simulink model "arducopter"  (R2021a)
settings: Solver=FixedStepAuto  StartTime=0.0  StopTime=sim.param.timeEnd  FixedStep=sim.param.dt  RelTol=1e-3
undefined symbols (not defined in the file or in its folder): DiscIntNeverNeededParam, sim
libraries: simulink x34, slident x4, vrlib x1
(part 6 of 8)

== system arducopter/Position Controller/set_pos_target_z_from_climb_rate()/input_vel_accel_z/calc accMin ==
  accMax : Inport
  Constant : Constant  Value=750  OutDataTypeStr=single
  Constant1 : Constant  Value=0  OutDataTypeStr=single
  Gain : Gain  Gain=-1
  Saturation Dynamic : simulink/Discontinuities/Saturation Dynamic  OutMin=[]  OutMax=[]  OutDataTypeStr=Inherit: Same as second input  OutDataType=fixdt(1, 16)  OutScaling=2^-10  DoSatur=off
  accMin : Outport
  wires:
  accMax/1 -> Saturation Dynamic/2
  Saturation Dynamic/1 -> Gain/1
  Gain/1 -> accMin/1
  Constant/1 -> Saturation Dynamic/1
  Constant1/1 -> Saturation Dynamic/3

== system arducopter/Position Controller/set_pos_target_z_from_climb_rate()/input_vel_accel_z/shape_vel_accel ==
  note: 1)
  note: shape_vel_accel()
      | Calculates the desired acceleration as a path from the current position, velocity and acceleration to an input velocity, considering the max velocity, acceleration and jerk.
      | Calculate KPa as time constant that defines the error decay in the kinematic path as the system approaches constant acceleration
      | Calculate the preliminary desired acceleration with the square root controller
      | Limit desired acceleration based on max. acceleration and jerk
  note: 3)
  note: 2)
  vel : Inport
  acc : Inport  Port=2
  velDes : Inport  Port=3
  accDes : Inport  Port=4
  accMin : Inport  Port=5
  accMax : Inport  Port=6
  jerkMax : Inport  Port=7
  dt : Inport  Port=8
  limitTotalAccel : Inport  Port=9
  MATLAB Function : MATLAB Function  TreatAsAtomicUnit=on
  Square Root Controller : MATLAB Function  TreatAsAtomicUnit=on
  calc_KPa : MATLAB Function  TreatAsAtomicUnit=on
  accDesShaped : Outport
  wires:
  vel/1 -> calc_KPa/1(velIn)
  acc/1 -> MATLAB Function/4(accIn)
  velDes/1 -> calc_KPa/2(vel)
  accMin/1 -> [accMin]
  accMax/1 -> [accMax]
  jerkMax/1 -> [jerkMax]
  dt/1 -> [dt]
  limitTotalAccel/1 -> MATLAB Function/8(limitTotalAccel)
  calc_KPa/2(KPa) -> Square Root Controller/2(p)
  Square Root Controller/1(correction_rate) -> MATLAB Function/1(accTar)
  MATLAB Function/1(accShaped) -> accDesShaped/1
  accDes/1 -> MATLAB Function/5(acc)
  calc_KPa/1(velErr) -> Square Root Controller/1(err)
  [dt] -> Square Root Controller/4(dt)
  [jerkMax] -> Square Root Controller/3(second_ord_lim)
  [jerkMax] -> calc_KPa/5(jerkMax)
  [dt] -> MATLAB Function/7(dt)
  [jerkMax] -> MATLAB Function/6(jerkMax)
  [accMin] -> calc_KPa/3(accMin)
  [accMax] -> calc_KPa/4(accMax)
  [accMin] -> MATLAB Function/2(accMin)
  [accMax] -> MATLAB Function/3(accMax)

== system arducopter/Position Controller/set_pos_target_z_from_climb_rate()/input_vel_accel_z/update_pos_vel_accel ==
  note: update_pos_vel_accel()
      | Single axis projection of position and velocity forwards in time based on
      | a time step of dt and acceleration off acc.
  posTarIn : Inport
  velDesIn : Inport  Port=2
  accDesIn : Inport  Port=3
  limitVectorZ : Inport  Port=4
  posErr : Inport  Port=5
  velErr : Inport  Port=6
  Constant : Constant  Value=sim.param.dt
  MATLAB Function : MATLAB Function  TreatAsAtomicUnit=on
  posTar : Outport
  velDes : Outport  Port=2
  wires:
  posTarIn/1 -> MATLAB Function/1(posIn)
  velDesIn/1 -> MATLAB Function/2(velIn)
  accDesIn/1 -> MATLAB Function/3(accIn)
  Constant/1 -> MATLAB Function/4(dt)
  MATLAB Function/1(pos) -> posTar/1
  limitVectorZ/1 -> MATLAB Function/5(limit)
  MATLAB Function/2(vel) -> velDes/1
  posErr/1 -> MATLAB Function/6(posErr)
  velErr/1 -> MATLAB Function/7(velErr)

== system arducopter/Rate Controller/PID Pitch Rate/Slew Limiter/Subsystem ==
  p_out : Inport
  d_out : Inport  Port=2
  ATC sample time : Constant  Value=sim.param.dt
  Add : Sum
  Divide : Product  Inputs=*/  OutDataTypeStr=single
  Subtract : Sum  Inputs=+-
  Unit Delay : UnitDelay  InitialCondition=sim.init.PIDP.P+sim.init.PIDP.D  SampleTime=-1  HasFrameUpgradeWarning=on
  sr_raw : Outport
  wires:
  ATC sample time/1 -> Divide/2
  Add/1 -> Unit Delay/1, Subtract/1
  Divide/1 -> sr_raw/1
  p_out/1 -> Add/1
  Unit Delay/1 -> Subtract/2
  Subtract/1 -> Divide/1
  d_out/1 -> Add/2

== system arducopter/Rate Controller/PID Roll Rate/Slew Limiter/Subsystem ==
  p_out : Inport
  d_out : Inport  Port=2
  ATC sample time : Constant  Value=sim.param.dt
  Add : Sum
  Divide : Product  Inputs=*/  OutDataTypeStr=single
  Subtract : Sum  Inputs=+-
  Unit Delay : UnitDelay  InitialCondition=sim.init.PIDR.P + sim.init.PIDR.D  SampleTime=-1  HasFrameUpgradeWarning=on
  sr_raw : Outport
  wires:
  ATC sample time/1 -> Divide/2
  Add/1 -> Unit Delay/1, Subtract/1
  Divide/1 -> sr_raw/1
  p_out/1 -> Add/1
  Unit Delay/1 -> Subtract/2
  Subtract/1 -> Divide/1
  d_out/1 -> Add/2

== system arducopter/Rate Controller/PID Yaw Rate/Slew Limiter/Subsystem ==
  p_out : Inport
  d_out : Inport  Port=2
  ATC sample time : Constant  Value=sim.param.dt
  Add : Sum
  Divide : Product  Inputs=*/  OutDataTypeStr=single
  Subtract : Sum  Inputs=+-
  Unit Delay : UnitDelay  InitialCondition=sim.init.PIDY.P+sim.init.PIDY.D  SampleTime=-1  HasFrameUpgradeWarning=on
  sr_raw : Outport
  wires:
  ATC sample time/1 -> Divide/2
  Add/1 -> Unit Delay/1, Subtract/1
  Divide/1 -> sr_raw/1
  p_out/1 -> Add/1
  Unit Delay/1 -> Subtract/2
  Subtract/1 -> Divide/1
  d_out/1 -> Add/2

== system arducopter/Attitude Controller/input_euler_angle_roll_pitch_euler_rate_yaw()/Feedforward enabled/input shaping/input shaping pitch angle ==
  note: AC_AttitudeControl::input_shaping_angle(float error_angle, float input_tc, float accel_max, float target_ang_vel, float desired_ang_vel, float max_ang_vel, float dt)
      | Calculation of velocity correction from an angle error. The angular velocity has acceleration and deceleration limits including basic jerk limiting using _input_tc.
      |
      | Function is called from input_shaping_angle(float error_angle, float smoothing_gain, float accel_max, float target_ang_vel, float dt) as input_shaping_angle(error_angle, smoothing_gain, accel_max, target_ang_vel, 0.0f, 0.0f, dt), so desired_ang_vel = 0 and max_ang_vel = 0
  pitchAngleErr : Inport
  pitchRateTarIn : Inport  Port=2
  pitchAccelMax : Inport  Port=3
  Constant : Constant  Value=sim.param.dt  VectorParams1D=off
  Constant1 : Constant  Value=sim.param.ATC.INPUT_TC  VectorParams1D=off
  Constant2 : Constant  Value=sim.param.dt  VectorParams1D=off
  Data Type Conversion : DataTypeConversion  OutDataTypeStr=single
  Data Type Conversion1 : DataTypeConversion  OutDataTypeStr=single
  MATLAB Function : MATLAB Function  TreatAsAtomicUnit=on
  MATLAB Function1 : MATLAB Function  TreatAsAtomicUnit=on
  Square Root Controller : MATLAB Function  TreatAsAtomicUnit=on
  calc p from input_tc : Subsystem
  eulerPitchRateTar : Outport
  wires:
  MATLAB Function1/1(eulerRateTar) -> eulerPitchRateTar/1
  [accelMax] -> MATLAB Function1/3(accelMax)
  [accelMax] -> Square Root Controller/3(second_ord_lim)
  Constant2/1 -> Data Type Conversion1/1
  Square Root Controller/1(correction_rate) -> MATLAB Function1/1(desiredAngVel)
  calc p from input_tc/1(p) -> Square Root Controller/2(p)
  Constant1/1 -> calc p from input_tc/1(input_tc)
  Constant/1 -> Data Type Conversion/1
  pitchAccelMax/1 -> [accelMax]
  MATLAB Function/1(radLim) -> Square Root Controller/1(err)
  pitchAngleErr/1 -> MATLAB Function/1(radIn)
  pitchRateTarIn/1 -> MATLAB Function1/2(targetAngVel)
  Data Type Conversion/1 -> Square Root Controller/4(dt)
  Data Type Conversion1/1 -> MATLAB Function1/4(dt)

== system arducopter/Attitude Controller/input_euler_angle_roll_pitch_euler_rate_yaw()/Feedforward enabled/input shaping/input shaping roll angle ==
  note: AC_AttitudeControl::input_shaping_angle(float error_angle, float input_tc, float accel_max, float target_ang_vel, float desired_ang_vel, float max_ang_vel, float dt)
      | Calculation of velocity correction from an angle error. The angular velocity has acceleration and deceleration limits including basic jerk limiting using _input_tc.
      |
      | Function is called from input_shaping_angle(float error_angle, float smoothing_gain, float accel_max, float target_ang_vel, float dt) as input_shaping_angle(error_angle, smoothing_gain, accel_max, target_ang_vel, 0.0f, 0.0f, dt), so desired_ang_vel = 0 and max_ang_vel = 0
  rollAngleErr : Inport
  rollRateTarIn : Inport  Port=2
  rollAccelMax : Inport  Port=3
  Constant : Constant  Value=sim.param.dt  VectorParams1D=off
  Constant1 : Constant  Value=sim.param.ATC.INPUT_TC  VectorParams1D=off
  Constant2 : Constant  Value=sim.param.dt  VectorParams1D=off
  Data Type Conversion : DataTypeConversion  OutDataTypeStr=single
  Data Type Conversion1 : DataTypeConversion  OutDataTypeStr=single
  MATLAB Function : MATLAB Function  TreatAsAtomicUnit=on
  MATLAB Function1 : MATLAB Function  TreatAsAtomicUnit=on
  Square Root Controller : MATLAB Function  TreatAsAtomicUnit=on
  calc p from input_tc : Subsystem
  eulerRollRateTar : Outport
  wires:
  rollAngleErr/1 -> MATLAB Function/1(radIn)
  MATLAB Function/1(radLim) -> Square Root Controller/1(err)
  rollAccelMax/1 -> [accelMax]
  Constant/1 -> Data Type Conversion/1
  Constant1/1 -> calc p from input_tc/1(input_tc)
  calc p from input_tc/1(p) -> Square Root Controller/2(p)
  Square Root Controller/1(correction_rate) -> MATLAB Function1/1(desiredAngVel)
  Constant2/1 -> Data Type Conversion1/1
  [accelMax] -> Square Root Controller/3(second_ord_lim)
  [accelMax] -> MATLAB Function1/3(accelMax)
  MATLAB Function1/1(eulerRateTar) -> eulerRollRateTar/1
  rollRateTarIn/1 -> MATLAB Function1/2(targetAngVel)
  Data Type Conversion/1 -> Square Root Controller/4(dt)
  Data Type Conversion1/1 -> MATLAB Function1/4(dt)

== system arducopter/Attitude Controller/input_euler_angle_roll_pitch_euler_rate_yaw()/Feedforward enabled/input shaping/input shaping yaw rate ==
  note: AC_AttitudeControl::input_shaping_ang_vel()
      | Limits the maximum acceleration resulting from the target yaw rate, so that the target yaw rate is slewed towards the input rate
  yawRateDes : Inport
  yawRateTar : Inport  Port=2
  eulerAccelMax : Inport  Port=3
  Constant2 : Constant  Value=sim.param.dt  VectorParams1D=off
  Data Type Conversion : DataTypeConversion  OutDataTypeStr=single
  MATLAB Function1 : MATLAB Function  TreatAsAtomicUnit=on
  eulerYawRateTar : Outport
  wires:
  yawRateDes/1 -> MATLAB Function1/1(desiredAngVel)
  Constant2/1 -> Data Type Conversion/1
  eulerAccelMax/1 -> MATLAB Function1/3(accelMax)
  MATLAB Function1/1(eulerRateTar) -> eulerYawRateTar/1
  yawRateTar/1 -> MATLAB Function1/2(targetAngVel)
  Data Type Conversion/1 -> MATLAB Function1/4(dt)

== system arducopter/Attitude Controller/input_euler_angle_roll_pitch_euler_rate_yaw()/thrust_heading_rotation_angles()/Yaw error limitation/Yaw limiting and recalculation of attitudeTarget ==
  note: Limit yaw error and calculate new attitudeTarget and attitudeError
  note: Create new attitudeError with limited yaw error
  note: Calculate new attitudeTarget with limited yawVecCorrection
  note: Limit yaw error based on maximum acceleration
  attitudeErrorIn : Inport
  thrustVecCorrection : Inport  Port=2
  attitudeBody : Inport  Port=3
  Enable : EnablePort
  Constant : Constant  Value=sim.param.ATC.ACCEL_Y_CONTROLLER_MAX_RADSS
  Constant1 : Constant  Value=sim.param.ATC.ANG_YAW_P
  Constant2 : Constant  Value=0  OutDataTypeStr=single
  Demux : Demux  Outputs=2
  Divide : Product  Inputs=*/
  Gain : Gain  Gain=-1
  MATLAB Function : MATLAB Function  TreatAsAtomicUnit=on
  MATLAB Function1 : MATLAB Function  TreatAsAtomicUnit=on
  MATLAB Function5 : MATLAB Function  TreatAsAtomicUnit=on
  MATLAB Function9 : MATLAB Function  TreatAsAtomicUnit=on
  MinMax : MinMax  Inputs=2
  MinMax1 : MinMax  Function=max  Inputs=2
  Mux : Mux  Inputs=3
  Mux1 : Mux  Inputs=3
  Selector : Selector  InputPortWidth=3  IndexOptions=Index vector (dialog)  Indices=[3]  OutputSizes=1
  Selector1 : Selector  InputPortWidth=3  IndexOptions=Index vector (dialog)  Indices=[1 2]  OutputSizes=1
  attitudeTarget : Outport
  attitudeError : Outport  Port=2
  wires:
  Constant/1 -> Divide/1
  Constant1/1 -> Divide/2
  [attitudeError] -> Selector/1
  Selector/1 -> MinMax/1
  Divide/1 -> MinMax/2, Gain/1
  MinMax/1 -> MinMax1/1
  Gain/1 -> MinMax1/2
  MinMax1/1 -> MATLAB Function/1(radIn)
  MATLAB Function/1(radLim) -> Mux1/3, Mux/3
  Constant2/1 -> Mux/2, Mux/1
  Mux/1 -> MATLAB Function5/1(vec)
  MATLAB Function5/1(q) -> MATLAB Function9/2(q2)  "yawVecCorrection"
  MATLAB Function9/1(qRes) -> MATLAB Function1/2(q2)
  thrustVecCorrection/1 -> MATLAB Function9/1(q1)
  attitudeBody/1 -> MATLAB Function1/1(q1)
  MATLAB Function1/1(qRes) -> attitudeTarget/1
  Mux1/1 -> attitudeError/1
  attitudeErrorIn/1 -> [attitudeError]
  [attitudeError] -> Selector1/1
  Selector1/1 -> Demux/1
  Demux/1 -> Mux1/1
  Demux/2 -> Mux1/2

== system arducopter/Attitude Controller/input_euler_angle_roll_pitch_euler_rate_yaw()/Feedforward enabled/input shaping/input shaping pitch angle/calc p from input_tc ==
  note: Calculation of proportional factor of square root controller.
      | Based on function argument of sqrt_controller() in AC_AttitudeControl::input_shaping_angle()
  input_tc : Inport
  Constant2 : Constant  Value=0.01  OutDataTypeStr=single
  Constant3 : Constant  OutDataTypeStr=single
  Divide : Product  Inputs=*/
  Max : MinMax  Function=max  Inputs=2
  p : Outport
  wires:
  Constant2/1 -> Max/2
  Max/1 -> Divide/2
  Constant3/1 -> Divide/1
  input_tc/1 -> Max/1
  Divide/1 -> p/1

== system arducopter/Attitude Controller/input_euler_angle_roll_pitch_euler_rate_yaw()/Feedforward enabled/input shaping/input shaping roll angle/calc p from input_tc ==
  note: Calculation of proportional factor of square root controller.
      | Based on function argument of sqrt_controller() in AC_AttitudeControl::input_shaping_angle()
  input_tc : Inport
  Constant2 : Constant  Value=0.01  OutDataTypeStr=single
  Constant3 : Constant  OutDataTypeStr=single
  Divide : Product  Inputs=*/
  Max : MinMax  Function=max  Inputs=2
  p : Outport
  wires:
  Constant2/1 -> Max/2
  Max/1 -> Divide/2
  Constant3/1 -> Divide/1
  input_tc/1 -> Max/1
  Divide/1 -> p/1

== matlab function arducopter/Position Controller/set z component of limit vec/MATLAB Function ==
function limVecZ = fcn(limLower, limUpper)
% Based on AC_PosControl::update_z_controller()

if limUpper
    limVecZ = single(1);
elseif limLower
    limVecZ = single(-1);
else
    limVecZ = single(0);
end

== matlab function arducopter/Throttle/Throttle Calculations/Throttle Hover/Throttle Hover Calculation ==
function thrHover = updateThrHov(dt, thrAct, zVelDes, zVelAct, thstHoverMax, thstHoverMin, thstHoverTC, thstHoverDefault, hoverLearn, thrMan)
%% Code is based on Copter::update_throttle_hover() in Attitude.cpp

global thrHoverAct;

% Use default throttle hover when throttle is set to manual
if (thrMan)
    thrHoverAct = thstHoverDefault;
end
if zVelDes > 0
    thrHoverAct = thstHoverDefault;
end

% Calc average throttle if we are in level hpver
if (thrAct > 0  && abs(zVelAct) < 60)
    %% Code is based on AP_MotorsMulticopter::update_throttle_hover(dt) in AP_MotorsMulticopter.cpp
    % Update throttle hover in dependency of the current output throttle
    if ( (hoverLearn ~= 0))
        thrHoverAct = thrHoverAct + (dt / (dt + thstHoverTC) ) * (thrAct - thrHoverAct);

        % Limit throttle hover to specified limits
        thrHoverAct = max( min( thrHoverAct, thstHoverMax), thstHoverMin);
    else % Set hover to default value if learning is disabled (AP_MotorsMulticopter.cpp)
        thrHoverAct = thstHoverDefault;
    end
end

thrHover = thrHoverAct;

== matlab function arducopter/Position Controller/set_pos_target_z_from_climb_rate()/input_vel_accel_z/shape_vel_accel/calc_KPa ==
function [velErr, KPa] = calcKPa(velIn, vel, accMin, accMax, jerkMax)
% First part of shape_vel_accel() in control.cpp
% Calculates correction gain KPa for the square root controller based on
% the jerk and acceleration limits.

% Velocity error to be corrected
velErr = velIn - vel;

% Calculate time constants and limits to ensure stable operation.
% The direction of acceleration limit is the same as the velocity error.
% This is because the velocity error is negative when slowing down while
% closing a positive position error.
if velErr > 0
    KPa = jerkMax / accMax;
else
    KPa = jerkMax / (-accMin);
end

== matlab function arducopter/Position Controller/set_pos_target_z_from_climb_rate()/input_vel_accel_z/shape_vel_accel/Square Root Controller ==
function correction_rate = sqrt_controller(err, p, second_ord_lim, dt)
% The square root controller
% Code is taken from sqrt_controller(...) in AC_PosControl.cpp.

if (second_ord_lim < 0 || second_ord_lim == 0)
   correction_rate = err * p;
elseif (p == 0)
    % P term is zero, but second order limit is positive
    if (err > 0)
        correction_rate = sqrt(single(2.0) * second_ord_lim * err);
    elseif (err < 0)
        correction_rate = sqrt(single(2.0) * second_ord_lim * -err);
    else
        correction_rate = single(0.0);
    end
else
    % P term and second order limit are positive, hence have been defined
    linear_dist = second_ord_lim / (p * p);
    % Check if error exceeds linear range of controller gain
    if (err > linear_dist)
        correction_rate = sqrt(single(2.0) * second_ord_lim * ( err - (linear_dist / single(2.0)) ));
    elseif (err < -linear_dist)
        correction_rate = -sqrt(single(2.0) * second_ord_lim * ( -err - (linear_dist / single(2.0)) ));
    else
        % Return linearly amplified correction if error is in linear range
        correction_rate = err * p;
    end
end

% Prevent oscillations by over-shooting the error correction in the last
% time step
if (dt ~= 0)
    correction_rate = max( min(correction_rate, abs(err) / dt), -abs(err) / dt);
end

== matlab function arducopter/Position Controller/set_pos_target_z_from_climb_rate()/input_vel_accel_z/shape_vel_accel/MATLAB Function ==
function accShaped = shapeAccelDes(accTar, accMin, accMax, accIn, acc, jerkMax, dt, limitTotalAccel)
% Second part of shape_vel_accel() in control.cpp
% Constrains desired acceleration based on acceleration limits and shapes
% kinematic path according to max jerk

%% 1) Limit desired acceleration based on acceleration limits
% Constrain correction acceleration from accMin to accMax
accTar = max(min(accTar, accMax), accMin);

% Velocity correction with input velocity
accTar = accTar + accIn;

% Constrain total acceleration from accMin to accMax
if limitTotalAccel
    accTar = max(min(accTar, accMax), accMin);
end

%% 2) Calculate required jerk limited adjustment to the current acceleration
% for the next time dt. Based on shape_accel()
accDelta = accTar - acc;
if jerkMax > 0
    accDelta = max(min(accDelta, jerkMax*dt), -jerkMax*dt);
end
accShaped = acc + accDelta;

== matlab function arducopter/Position Controller/get_pilot_speed_dn()/MATLAB Function ==
function dnMax = getPilotSpeedDown(dnMaxIn, upMax)
% Get maximum vertical descending velocity. Called in ModeAltHold::init()
% in the function call for AC_PosControl::set_max_speed_accel_z()
if dnMaxIn == 0
    dnMax = abs(upMax);
else
    dnMax = abs(dnMaxIn);
end

== matlab function arducopter/Throttle/Throttle Calculations/Throttle Limiting based on battery state/Update Lift Max from Battery Voltage ==
function [battVoltFilt, liftMax, battVoltMinAct, battVoltRestEstAct] = fcn(battVoltFiltLast, battVoltRestEst, battVoltMax, battVoltMin, thstCurveExpo, loop_rate)
% Code taken from AP_MotorsMulticopter::update_lift_max_from_batt_voltage()
% in AP_MotorsMulticopter.cpp

% Check if batt_volt_min is too small
if (battVoltMax <= 0 || (battVoltMin >= battVoltMax) ...
        || battVoltRestEst < 0.25 * battVoltMin)
    battVoltFilt = single(1.0);
    liftMax = single(1.0);
    battVoltMinAct = battVoltMin;
    battVoltRestEstAct = battVoltRestEst;
    return;
end

% Set lower battery voltage limit for thrust scaling to a new value
battVoltMinAct = max(battVoltMin, battVoltMax * 0.6);

% Constrain resting voltage estimate (resting voltage is actual voltage
% with sag removed based on current draw and resistance)
battVoltRestEstAct = max( min(battVoltRestEst, battVoltMax), battVoltMin);

%% Filter battery voltage at 0.5 Hz. 
% Cutoff Frequency defined in AP_MotorsMulticopter.h
cutoff_freq = single(0.5);
% Calculate time constant and alpha value
T = 1 / (2 * pi * cutoff_freq);
dt = 1 / loop_rate;
alpha = dt / (dt + T);
alpha = max( min( alpha, 1.0), 0.0);

% Filter input is batt_volt_rest_est / batt_volt_comp_max
in = battVoltRestEstAct / battVoltMax;

% Output calculation
battVoltFilt = battVoltFiltLast + (in - battVoltFiltLast) * alpha;

%% Calculate lift_max
thstCurveExpo = max( min(thstCurveExpo, 1), -1);
liftMax = battVoltFilt * (1 - thstCurveExpo) + thstCurveExpo * battVoltFilt * battVoltFilt;

== matlab function arducopter/Throttle/Throttle Calculations/Throttle Limiting based on battery state/Get current throttle limit ==
function [thrThstMax, thrLimit] = getCurrentLimitMaxThrottle(batVoltMin, batCurrMax, batCurrT, loop_rate, batCurr, batRes, batVolt, thrHover, thrLimitLast)
% Code is based on AP_MotorsMulticopter::get_current_limit_max_throttle()
% in AP_MotorsMulticopter.cpp. 
% Returns a throttle limit based on the maximum battery current as a number
% from 0~1 in the range throttle_min to throttle_max.

% Return maximum if current limiting is disabled
if(batCurrMax <= 0) 
    thrLimit = single(1.0);
    thrThstMax = single(1.0);
    return;
end
% Return maximum if battery resistance is not measured
if(batRes == 0)
    thrLimit = single(1.0);
    thrThstMax = single(1.0);
    return;
end

%% Calculate throttle limit
% The throttle limit represents the maximum throttle potential that is left
% based on the actual current compared to the maximum battery current.

% Maximum current to prevent voltage sag below batt_voltage_min
% Since the actual battery current level is used as the minimum for the limit,
% the actual current can still be used to maintain the current throttle. 
batt_curr_max_new = min(batCurrMax, batCurr + (batVolt - batVoltMin) / batRes);
% Calcualte current artion
batt_curr_ratio = batCurr / batt_curr_max_new;
% Calculate time step
dt = 1 / loop_rate;
% Calculate throttle limit as the additional throttle on top of throttle
% hover
thrLimit = thrLimitLast + (dt / (dt + batCurrT)) * (1.0 - batt_curr_ratio);
% Throttle limit drops to 20% between hover an full throttle
thrLimit = max( min( thrLimit, 1.0), 0.2);

% Calculate maximum throttle as sum of hover throttle and the possible
% additional throttle based on the maximum current.
thrThstMax = thrHover + ((1.0 - thrHover) * thrLimit);

== matlab function arducopter/Rate Controller/PID Yaw Rate/I/Integrator ==
function integrator_out = fcn(error, integrator, limit_flg, ki, i_max, dt)
% Code is based on AC_PID::update_i() in AC_PID.cpp.

% Check plausibility of input parameters
if (ki ~= 0 && dt > 0)
    % Only allow integration if limit is not set or the absolute sum of the
    % integrator would be reduced.
    if (~limit_flg || (integrator > 0 && error < 0) || (integrator < 0 && error > 0))
        integrator_out = integrator + error * ki * dt;
        integrator_out = max( min(integrator_out, i_max), -i_max);
    else % Otherwise, keep old integrator value
        integrator_out = integrator;
    end
else % Reset integrator if input parameters are not plausible
    integrator_out = single(0.0);
end

== matlab function arducopter/Rate Controller/PID Roll Rate/I/Integrator ==
function integrator_out = fcn(error, integrator, limit_flg, ki, i_max, dt)
% Code is based on AC_PID::update_i() in AC_PID.cpp.

% Check plausibility of input parameters
if (ki ~= 0 && dt > 0)
    % Only allow integration if limit is not set or the absolute sum of the
    % integrator would be reduced.
    if (~limit_flg || (integrator > 0 && error < 0) || (integrator < 0 && error > 0))
        integrator_out = integrator + error * ki * dt;
        integrator_out = max( min(integrator_out, i_max), -i_max);
    else % Otherwise, keep old integrator value
        integrator_out = integrator;
    end
else % Reset integrator if input parameters are not plausible
    integrator_out = single(0.0);
end

== matlab function arducopter/Throttle/Throttle Calculations/Get compensation gain ==
function compGain = fcn(liftMax, airDensityRatio)
% Code is based on AP_MotorsMulticopter::get_compensation_gain() in
% AP_MotorsMulticopter.cpp.

% Avoid to divide by zero
if(liftMax <= 0.0)
    compGain = single(1.0);
    return;
end

compGain = 1.0 / liftMax;

% Limit air density ratio
airDensityRatioLim = double(max( min( airDensityRatio, 1.25 ), 0.5));

if (airDensityRatio > 0.3 && airDensityRatio < 1.5)
   compGain = compGain * (1.0 / airDensityRatioLim); 
end

== matlab function arducopter/Rate Controller/PID Roll Rate/Slew Limiter/Calculate Dmod ==
function Dmod   = fcn(slew_rate, sr_max, sr_tau, dt, time)
% Code is based on SlewLimiter::modifier() in SlewLimiter.cpp. 

% Define global variables, so that quanitities do not have to be fed back
% to the function
global pos_event_stored;
global pos_event_idx;
global pos_event_ms;
global max_pos_slew_rate;
global max_pos_slew_event_ms;
global neg_event_stored;
global neg_event_idx;
global neg_event_ms;
global max_neg_slew_rate;
global max_neg_slew_event_ms;
global modifier_slew_rate;
global output_slew_rate;

% Definition of constants as done in SlewLimiter.h
N_EVENTS = uint32(3); % Number of positive and negative consecutive slew rate exceedance events recorded. Set to 3 because of 1-based indexing.
WINDOW_MS = uint32(300); % Time in ms required for half a cycle of the slowest oscillation frequency expected
MODIFIER_GAIN = 1.5; % Ratio of modifier reduction to slew rate exceedance

% Check if slew limiter is activated
if(sr_max <= 0)
   Dmod = single(1.0);
end

now_ms = uint32(time);
decay_alpha = min(dt, sr_tau) / sr_tau;

%% Save exceedance events in event time vector
% Store a series of positive slew rate exceedance events
if (~pos_event_stored && slew_rate > sr_max)
    if (pos_event_idx >= N_EVENTS)
        pos_event_idx(:) = 1;
    end
    pos_event_ms(pos_event_idx) = now_ms;
    pos_event_idx(:) = pos_event_idx + 1;
    pos_event_stored = true;
    neg_event_stored = false;
end

% Store a series of negative slew rate exceedance events
if (~neg_event_stored && slew_rate < -sr_max)
    if (neg_event_idx >= N_EVENTS)
        neg_event_idx(:) = 1;
    end
    neg_event_ms(neg_event_idx) = now_ms;
    neg_event_idx(:) = neg_event_idx + 1;
    pos_event_stored = false;
    neg_event_stored = true;
end

% Find oldest event time
oldest_ms = now_ms;
for i=1:N_EVENTS-1
   if (pos_event_ms(i) < oldest_ms)
       oldest_ms = pos_event_ms(i);
   end
   if (neg_event_ms(i) < oldest_ms)
       oldest_ms = neg_event_ms(i);
   end
end

%% Calculate maximum slew rate
% Save new maximum slew rates, if oldest maximum is exceeded
% OR decay the peak slew rates (pos. and neg.) if they are outside the
% observed time window
if (slew_rate > max_pos_slew_rate)
    max_pos_slew_rate(:) = min(slew_rate, 10 * sr_max);
    max_pos_slew_event_ms = now_ms;
elseif (now_ms - max_pos_slew_event_ms > WINDOW_MS)
    max_pos_slew_rate = max_pos_slew_rate * (1.0 - decay_alpha);
end

if (slew_rate < -max_neg_slew_rate)
    max_neg_slew_rate(:) = min(-slew_rate, 10 * sr_max);
    max_neg_slew_event_ms = now_ms;
elseif (now_ms - max_neg_slew_event_ms > WINDOW_MS)
    max_neg_slew_rate = max_neg_slew_rate * (1.0 - decay_alpha);
end

% Calculate the averaged maximum slew rate
raw_slew_rate = 0.5 * (max_pos_slew_rate + max_neg_slew_rate);

% When the oldest exceedance event falls outside of the window required for
% the number of exceedance events, apply a further reduction to the maximum
% slew rate. This prevents unwanted gain reductions caused by spikes in the
% demanded angular rates due to changed control modes or similar causes.
modifier_input = raw_slew_rate;
if(now_ms - oldest_ms > N_EVENTS * WINDOW_MS) % no incrementation of N_EVENTS because of 1 based indexing
   oldest_time_from_window = single(0.001) * single(now_ms - oldest_ms - N_EVENTS * WINDOW_MS); 
   modifier_input = modifier_input * single(exp(-oldest_time_from_window / sr_tau));
end

%% Calculation of modifier and output slew rate

% Apply filter to slew rate in order to reduce effects of large setpoint
% changes
attack_alpha = min(2.0 * decay_alpha, 1.0);

modifier_slew_rate = modifier_slew_rate + (modifier_input - modifier_slew_rate) * attack_alpha;
modifier_slew_rate = min(modifier_slew_rate, modifier_input);

output_slew_rate = output_slew_rate + (raw_slew_rate - output_slew_rate) * attack_alpha;
output_slew_rate = min(raw_slew_rate, output_slew_rate);

% Calculate modifier. Only has an impact if sr_max is exceeded by averaged
% slew rate.
if(modifier_slew_rate > sr_max)
    Dmod(:) = sr_max / (sr_max + MODIFIER_GAIN * (modifier_slew_rate - sr_max));
else
    Dmod(:) = 1.0;
end

== matlab function arducopter/Rate Controller/PID Roll Rate/Slew Limiter/Lowpass Filter ==
function out  = fcn(in, cutoff_freq, loop_rate, out_last)
% The code is based on the apply(sample, cutoff_freq, dt) function in
% LowPassFilter.cpp
dt = 1 / loop_rate;

% Check if filter is supposed to be filtering
if (cutoff_freq <=0 || dt <= 0)
    out = in;
    return;
end

% Calculate time constant and alpha value
T = 1 / (2 * pi * cutoff_freq);
alpha = dt / (dt + T);
alpha = max( min( alpha, 1.0), 0.0);

% Output calculation
out = out_last + (in - out_last) * alpha;

== matlab function arducopter/Throttle/Throttle Calculations/Air density Calculation/Get equivalent to true airspeed EAS2TAS ==
function eas2tas = fcn(alt, airPress, gndTemp)
% Code is based on AP_Baro::get_EAS2TAS() in AP_Baro.cpp.

% Constants
C_TO_KELVIN = single(273.15); % Conversion offset from celsius to kelvin
ISA_LAPSE_RATE = single(0.0065);
ISA_GAS_CONSTANT = single(287.26);
SSL_AIR_DENSITY = single(1.225);

% Global variables
global EAS2TAS;
global last_alt_EAS2TAS;

% Check if altitude has changed significally
if ((abs(alt - last_alt_EAS2TAS) < 25.0) && EAS2TAS ~= 0)
    % Change too small to require re-calculating
   eas2tas = EAS2TAS;
   return;
end

if (airPress == 0)
   eas2tas = single(1.0);
   return;
end

tempK = single(gndTemp + C_TO_KELVIN - ISA_LAPSE_RATE * alt);
eas2tas_squared = SSL_AIR_DENSITY / (airPress / (ISA_GAS_CONSTANT * tempK));
if (eas2tas_squared <= 0)
    eas2tas = single(1.0);
    return;
end
EAS2TAS = sqrt(eas2tas_squared);
last_alt_EAS2TAS = alt;
eas2tas = EAS2TAS;

== matlab function arducopter/Throttle/Throttle Calculations/Air density Calculation/Get air density ratio ==
function airDensityRatio = fcn(eas2tas)
% Code is based on AP_Baro::get_air_density_ratio() in AP_Baro.cpp.
if (eas2tas > 0.0)
    airDensityRatio = single(1.0 / (eas2tas*eas2tas));
else
    airDensityRatio = single(1.0);
end

== matlab function arducopter/Attitude Controller/input_euler_angle_roll_pitch_euler_rate_yaw()/Feedforward enabled/input shaping/input shaping pitch angle/MATLAB Function1 ==
function eulerRateTar = input_shaping_ang_vel(desiredAngVel, targetAngVel, accelMax, dt)
% Limits acceleration and deceleration of a velocity request
% Code based on AC_AttitudeControl::input_shaping_ang_vel()

% Acceleration is limited directly to smooth the beginning of the curve
if accelMax > 0
    deltaAngVel = accelMax * dt;
    eulerRateTar = min(max(desiredAngVel, targetAngVel - deltaAngVel), targetAngVel + deltaAngVel);
else
    eulerRateTar = desiredAngVel;
end

== matlab function arducopter/Attitude Controller/input_euler_angle_roll_pitch_euler_rate_yaw()/Feedforward enabled/input shaping/input shaping yaw rate/MATLAB Function1 ==
function eulerRateTar = input_shaping_ang_vel(desiredAngVel, targetAngVel, accelMax, dt)
% Limits acceleration and deceleration of a velocity request
% Code based on AC_AttitudeControl::input_shaping_ang_vel()

% Acceleration is limited directly to smooth the beginning of the curve
if accelMax > 0
    deltaAngVel = accelMax * dt;
    eulerRateTar = min(max(desiredAngVel, targetAngVel - deltaAngVel), targetAngVel + deltaAngVel);
else
    eulerRateTar = desiredAngVel;
end

== matlab function arducopter/Rate Controller/PID Yaw Rate/Slew Limiter/Calculate Dmod ==
function Dmod   = fcn(slew_rate, sr_max, sr_tau, dt, time)
% Code is based on SlewLimiter::modifier() in SlewLimiter.cpp. 

% Define global variables, so that quanitities do not have to be fed back
% to the function
global pos_event_stored;
global pos_event_idx;
global pos_event_ms;
global max_pos_slew_rate;
global max_pos_slew_event_ms;
global neg_event_stored;
global neg_event_idx;
global neg_event_ms;
global max_neg_slew_rate;
global max_neg_slew_event_ms;
global modifier_slew_rate;
global output_slew_rate;

% Definition of constants as done in SlewLimiter.h
N_EVENTS = uint32(3); % Number of positive and negative consecutive slew rate exceedance events recorded. Set to 3 because of 1-based indexing.
WINDOW_MS = uint32(300); % Time in ms required for half a cycle of the slowest oscillation frequency expected
MODIFIER_GAIN = 1.5; % Ratio of modifier reduction to slew rate exceedance

% Check if slew limiter is activated
if(sr_max <= 0)
   Dmod = single(1.0);
end

now_ms = uint32(time);
decay_alpha = min(dt, sr_tau) / sr_tau;

%% Save exceedance events in event time vector
% Store a series of positive slew rate exceedance events
if (~pos_event_stored && slew_rate > sr_max)
    if (pos_event_idx >= N_EVENTS)
        pos_event_idx(:) = 1;
    end
    pos_event_ms(pos_event_idx) = now_ms;
    pos_event_idx(:) = pos_event_idx + 1;
    pos_event_stored = true;
    neg_event_stored = false;
end

% Store a series of negative slew rate exceedance events
if (~neg_event_stored && slew_rate < -sr_max)
    if (neg_event_idx >= N_EVENTS)
        neg_event_idx(:) = 1;
    end
    neg_event_ms(neg_event_idx) = now_ms;
    neg_event_idx(:) = neg_event_idx + 1;
    pos_event_stored = false;
    neg_event_stored = true;
end

% Find oldest event time
oldest_ms = now_ms;
for i=1:N_EVENTS-1
   if (pos_event_ms(i) < oldest_ms)
       oldest_ms = pos_event_ms(i);
   end
   if (neg_event_ms(i) < oldest_ms)
       oldest_ms = neg_event_ms(i);
   end
end

%% Calculate maximum slew rate
% Save new maximum slew rates, if oldest maximum is exceeded
% OR decay the peak slew rates (pos. and neg.) if they are outside the
% observed time window
if (slew_rate > max_pos_slew_rate)
    max_pos_slew_rate(:) = min(slew_rate, 10 * sr_max);
    max_pos_slew_event_ms = now_ms;
elseif (now_ms - max_pos_slew_event_ms > WINDOW_MS)
    max_pos_slew_rate = max_pos_slew_rate * (1.0 - decay_alpha);
end

if (slew_rate < -max_neg_slew_rate)
    max_neg_slew_rate(:) = min(-slew_rate, 10 * sr_max);
    max_neg_slew_event_ms = now_ms;
elseif (now_ms - max_neg_slew_event_ms > WINDOW_MS)
    max_neg_slew_rate = max_neg_slew_rate * (1.0 - decay_alpha);
end

% Calculate the averaged maximum slew rate
raw_slew_rate = 0.5 * (max_pos_slew_rate + max_neg_slew_rate);

% When the oldest exceedance event falls outside of the window required for
% the number of exceedance events, apply a further reduction to the maximum
% slew rate. This prevents unwanted gain reductions caused by spikes in the
% demanded angular rates due to changed control modes or similar causes.
modifier_input = raw_slew_rate;
if(now_ms - oldest_ms > N_EVENTS * WINDOW_MS) % no incrementation of N_EVENTS because of 1 based indexing
   oldest_time_from_window = single(0.001) * single(now_ms - oldest_ms - N_EVENTS * WINDOW_MS); 
   modifier_input = modifier_input * single(exp(-oldest_time_from_window / sr_tau));
end

%% Calculation of modifier and output slew rate

% Apply filter to slew rate in order to reduce effects of large setpoint
% changes
attack_alpha = min(2.0 * decay_alpha, 1.0);

modifier_slew_rate = modifier_slew_rate + (modifier_input - modifier_slew_rate) * attack_alpha;
modifier_slew_rate = min(modifier_slew_rate, modifier_input);

output_slew_rate = output_slew_rate + (raw_slew_rate - output_slew_rate) * attack_alpha;
output_slew_rate = min(raw_slew_rate, output_slew_rate);

% Calculate modifier. Only has an impact if sr_max is exceeded by averaged
% slew rate.
if(modifier_slew_rate > sr_max)
    Dmod(:) = sr_max / (sr_max + MODIFIER_GAIN * (modifier_slew_rate - sr_max));
else
    Dmod(:) = 1.0;
end

== matlab function arducopter/Rate Controller/PID Yaw Rate/Slew Limiter/Lowpass Filter ==
function out  = fcn(in, cutoff_freq, loop_rate, out_last)
% The code is based on the apply(sample, cutoff_freq, dt) function in
% LowPassFilter.cpp
dt = 1 / loop_rate;

% Check if filter is supposed to be filtering
if (cutoff_freq <=0 || dt <= 0)
    out = in;
    return;
end

% Calculate time constant and alpha value
T = 1 / (2 * pi * cutoff_freq);
alpha = dt / (dt + T);
alpha = max( min( alpha, 1.0), 0.0);

% Output calculation
out = out_last + (in - out_last) * alpha;

== matlab function arducopter/Position Controller/PID Velocity z/I/Integrator ==
function integrator_out = fcn(error, integrator, limitNeg, limitPos, ki, i_max, dt)
% Code is based on AC_PID_Basic::update_i() in AC_PID_Basic.

% Check plausibility of input parameters
if (ki ~= 0)
    % Integration can only be executed if limits are not exceeded or if
    % limits are exceeded but the current error would reduce output
    if (~((limitNeg && error < 0) || (limitPos && error > 0)))
        integrator_out = integrator + error * ki * dt;
        integrator_out = max( min(integrator_out, i_max), -i_max);
    else % Otherwise, keep old integrator value
        integrator_out = integrator;
    end
else % Reset integrator if input parameters are not plausible
    integrator_out = single(0.0);
end

== matlab function arducopter/Position Controller/PID Acceleration z/I/Integrator ==
function integrator_out = fcn(error, integrator, limit_flg, ki, i_max, dt)
% Code is based on AC_PID::update_i() in AC_PID, line 230.

% Check plausibility of input parameters
if (ki ~= 0 && dt > 0)
    % Only allow integration if limit is not set or the absolute sum of the
    % integrator would be reduced.
    if (~limit_flg || (integrator > 0 && error < 0) || (integrator < 0 && error > 0))
        integrator_out = integrator + error * ki * dt;
        integrator_out = max( min(integrator_out, i_max), -i_max);
    else % Otherwise, keep old integrator value
        integrator_out = integrator;
    end
else % Reset integrator if input parameters are not plausible
    integrator_out = single(0.0);
end

== matlab function arducopter/Position Controller/PID Acceleration z/Slew Limiter/Calculate Dmod ==
function Dmod   = fcn(slew_rate, sr_max, sr_tau, dt, time)
% Code is based on SlewLimiter::modifier() in SlewLimiter.cpp. 

% Define global variables, so that quanitities do not have to be fed back
% to the function
global pos_event_stored;
global pos_event_idx;
global pos_event_ms;
global max_pos_slew_rate;
global max_pos_slew_event_ms;
global neg_event_stored;
global neg_event_idx;
global neg_event_ms;
global max_neg_slew_rate;
global max_neg_slew_event_ms;
global modifier_slew_rate;
global output_slew_rate;

% Definition of constants as done in SlewLimiter.h
N_EVENTS = uint32(3); % Number of positive and negative consecutive slew rate exceedance events recorded. Set to 3 because of 1-based indexing.
WINDOW_MS = uint32(300); % Time in ms required for half a cycle of the slowest oscillation frequency expected
MODIFIER_GAIN = 1.5; % Ratio of modifier reduction to slew rate exceedance

% Check if slew limiter is activated
if(sr_max <= 0)
   Dmod = single(1.0);
end

now_ms = uint32(time);
decay_alpha = min(dt, sr_tau) / sr_tau;

%% Save exceedance events in event time vector
% Store a series of positive slew rate exceedance events
if (~pos_event_stored && slew_rate > sr_max)
    if (pos_event_idx >= N_EVENTS)
        pos_event_idx(:) = 1;
    end
    pos_event_ms(pos_event_idx) = now_ms;
    pos_event_idx(:) = pos_event_idx + 1;
    pos_event_stored = true;
    neg_event_stored = false;
end

% Store a series of negative slew rate exceedance events
if (~neg_event_stored && slew_rate < -sr_max)
    if (neg_event_idx >= N_EVENTS)
        neg_event_idx(:) = 1;
    end
    neg_event_ms(neg_event_idx) = now_ms;
    neg_event_idx(:) = neg_event_idx + 1;
    pos_event_stored = false;
    neg_event_stored = true;
end

% Find oldest event time
oldest_ms = now_ms;
for i=1:N_EVENTS-1
   if (pos_event_ms(i) < oldest_ms)
       oldest_ms = pos_event_ms(i);
   end
   if (neg_event_ms(i) < oldest_ms)
       oldest_ms = neg_event_ms(i);
   end
end

%% Calculate maximum slew rate
% Save new maximum slew rates, if oldest maximum is exceeded
% OR decay the peak slew rates (pos. and neg.) if they are outside the
% observed time window
if (slew_rate > max_pos_slew_rate)
    max_pos_slew_rate(:) = min(slew_rate, 10 * sr_max);
    max_pos_slew_event_ms = now_ms;
elseif (now_ms - max_pos_slew_event_ms > WINDOW_MS)
    max_pos_slew_rate = max_pos_slew_rate * (1.0 - decay_alpha);
end

if (slew_rate < -max_neg_slew_rate)
    max_neg_slew_rate(:) = min(-slew_rate, 10 * sr_max);
    max_neg_slew_event_ms = now_ms;
elseif (now_ms - max_neg_slew_event_ms > WINDOW_MS)
    max_neg_slew_rate = max_neg_slew_rate * (1.0 - decay_alpha);
end

% Calculate the averaged maximum slew rate
raw_slew_rate = 0.5 * (max_pos_slew_rate + max_neg_slew_rate);

% When the oldest exceedance event falls outside of the window required for
% the number of exceedance events, apply a further reduction to the maximum
% slew rate. This prevents unwanted gain reductions caused by spikes in the
% demanded angular rates due to changed control modes or similar causes.
modifier_input = raw_slew_rate;
if(now_ms - oldest_ms > N_EVENTS * WINDOW_MS) % no incrementation of N_EVENTS because of 1 based indexing
   oldest_time_from_window = single(0.001) * single(now_ms - oldest_ms - N_EVENTS * WINDOW_MS); 
   modifier_input = modifier_input * single(exp(-oldest_time_from_window / sr_tau));
end

%% Calculation of modifier and output slew rate

% Apply filter to slew rate in order to reduce effects of large setpoint
% changes
attack_alpha = min(2.0 * decay_alpha, 1.0);

modifier_slew_rate = modifier_slew_rate + (modifier_input - modifier_slew_rate) * attack_alpha;
modifier_slew_rate = min(modifier_slew_rate, modifier_input);

output_slew_rate = output_slew_rate + (raw_slew_rate - output_slew_rate) * attack_alpha;
output_slew_rate = min(raw_slew_rate, output_slew_rate);

% Calculate modifier. Only has an impact if sr_max is exceeded by averaged
% slew rate.
if(modifier_slew_rate > sr_max)
    Dmod(:) = sr_max / (sr_max + MODIFIER_GAIN * (modifier_slew_rate - sr_max));
else
    Dmod(:) = 1.0;
end

== matlab function arducopter/Motor Mixer/Calculate motor thrust ==
function [limitRoll, limitPitch, limitYaw, limitThrLower, limitThrUpper, thrOut, thstOut] = outputArmedStabilizing(roll, pitch, yaw, thrIn, thrAvgMax, thrThstMaxIn, compGain, yawHeadroom, numMotors, facMotors)
% The calculation is taken from output_armed_stabilizing() in
% AP_MotorsMatrix.cpp.
% Contrary to the original code, lost motors are not considered

global thst_rpyt;

%% Preperations
% Definitions
roll_factor = facMotors(1,:);              % Factors of motors for thrust on differen axis - needs to moved to Init-file, together with calculation
pitch_factor = facMotors(2,:);
yaw_factor = facMotors(3,:);
throttle_factor = facMotors(4,:);
limitRoll = false;                             % Initialize limit flags to prevent missing assignment error of Simulink
limitPitch = false;
limitYaw = false;
limitThrLower = false;
limitThrUpper = false;
yaw_allowed = single(1.0);                          % Amount of yaw that can be realized
rpy_scale = single(1.0);                            % Scale factor to fit roll, pitch and yaw within motor limits
throttle_thrust_best_rpy = single(0.0);             % Amount of throttle that provides maximum roll, pitch and yaw without climbing                      
thrust_boost_ratio = single(0.0);                   % Ratio for thrust boosting in case of a motor failure. Set to 0 for normal operation!     

% TODO: Voltage and air pressure compensation
roll_thrust = roll * compGain;
pitch_thrust = pitch * compGain;
yaw_thrust = yaw * compGain;
throttle_thrust = thrIn * compGain;             % Pilot's desired throttle
thrAvgMax = thrAvgMax * compGain;

% Calculate maximum throttle thrust input value
throttle_thrust_max = thrust_boost_ratio + (1.0 - thrust_boost_ratio) * thrThstMaxIn;

% Sanity check: Throttle above zero and below current limnited throttle.
% Limit Throttle otherwise
if (throttle_thrust <= 0)
    throttle_thrust = single(0.0);
    limitThrLower = true;
end
if (throttle_thrust >= throttle_thrust_max)
    throttle_thrust = throttle_thrust_max;
    limitThrUpper = true;
end
% Limit throttle average max
thrAvgMax = max( min( thrAvgMax, throttle_thrust_max), throttle_thrust);
% Calculate highest allowed average throttle that will provide maximum
% control range of roll, pitch and yaw without climbing
throttle_thrust_best_rpy = min(single(0.5), thrAvgMax);

%% Calculation of the throttle that gives most room for yaw
% This corresponds to the lower of
%   1. 0.5 - (rpy_low + rpy_high) / 2.0) --> This gives the maximum
%   possible margin above the highest motor and below the lowest
%   2. The higher of
%       a) Pilots throttle input
%       b) The point throttle_rpy_mix between pilot's input throttle and
%       hover throttle

% First: Calculate amount of yaw that fits into throttle range
rp_low = single(1.0);
rp_high = single(-1.0);
for i=1:numMotors
    % Combined thrust output of roll and pitch
    thst_rpyt(i) = roll_thrust * roll_factor(i) + pitch_thrust * pitch_factor(i); 
    
    % Record lowest thrust command
    if (thst_rpyt(i) < rp_low)
        rp_low = thst_rpyt(i);
    end
    % Record highest thrust command
    if (thst_rpyt(i) > rp_high)
        rp_high = thst_rpyt(i);
    end
    
    % Check maximum yaw control that can be used
    if(yaw_factor(i)~=0)
        if ((yaw_thrust * yaw_factor(i)) > 0)
           yaw_allowed = min(yaw_allowed, abs( max(1.0 - throttle_thrust_best_rpy + thst_rpyt(i), 0.0)/yaw_factor(i) ) ); 
        else
           yaw_allowed = min(yaw_allowed, abs( max(throttle_thrust_best_rpy + thst_rpyt(i), 0.0)/yaw_factor(i) ) );
        end
    end    
end

% Calculate the maximum yaw control that can be used
yaw_allowed_min = yawHeadroom / 1000.0;
% If thrust boost is enabled, increase headroom to 50%
yaw_allowed_min = thrust_boost_ratio * 0.5 + (1.0 - thrust_boost_ratio) * yaw_allowed_min;

yaw_allowed = max(yaw_allowed, yaw_allowed_min);

%% Add yaw control to thrust outputs
% Limit yaw thrust to allowed range
if (abs(yaw_thrust) > yaw_allowed)
    yaw_thrust = min( max(-yaw_allowed, yaw_thrust), yaw_allowed);
    limitYaw = true;
end

rpy_low = single(1.0);
rpy_high = single(-1.0);
for i=1:numMotors
    % Combined thrust command for roll, pitch and yaw
   thst_rpyt(i) = thst_rpyt(i) + yaw_thrust * yaw_factor(i);
   
   % Record lowest thrust command
    if (thst_rpyt(i) < rpy_low)
        rpy_low = thst_rpyt(i);
    end
    % Record highest thrust command
    if (thst_rpyt(i) > rpy_high)
        rpy_high = thst_rpyt(i);
    end
end

%% Scale outputs
% Calculate any sclaing that is needed to fit combined thrust outputs
% within the output range
if (rpy_high - rpy_low > 1.0)
    rpy_scale(:) = 1.0 / (rpy_high-rpy_low);
end
if (thrAvgMax + rpy_low < 0)
    rpy_scale(:) = min(rpy_scale, -thrAvgMax / rpy_low);
end

% Calculate how close the motors can come to the desired throttle
rpy_high = rpy_high * rpy_scale;
rpy_low = rpy_low * rpy_scale;
throttle_thrust_best_rpy = -rpy_low;
% Calculate the difference between pilot's desired throttle and
% throttle_thrust_best_rpy
thr_adj = single(throttle_thrust - throttle_thrust_best_rpy);
if (rpy_scale < 1.0) % Full range of throttle is already being used
    limitRoll(:) = true;
    limitPitch(:) = true;
    limitYaw(:) = true;
    if (thr_adj > 0.0)
       limitThrUpper = true; 
    end
    thr_adj(:) = 0.0;
else
    if (thr_adj < 0.0) % Throttle can't be reduced to reach desired value
        thr_adj(:) = 0.0;
    elseif (thr_adj > 1.0 - (throttle_thrust_best_rpy + rpy_high))
       % Throttle can't be increased to desired value
       thr_adj(:) = 1.0 - (throttle_thrust_best_rpy + rpy_high);
       limitThrUpper = true;
    end
end

%% Calculate resulting thrust outputs
% Calculate adjusted throttle value
throttle_thrust_best_plus_adj = throttle_thrust_best_rpy + thr_adj;
% Add scaled roll, pitch, constrained yaw and throttle for each motor
for i=1:numMotors
    % Combined thrust is the sum of the maximum possible desired throttle
    % "throttle_thrust_best_plus_adj" and the needed thrust to realize the
    % desired angular motion "thrust_rpyt_out(i)"
    thst_rpyt(i) = (throttle_thrust_best_plus_adj * throttle_factor(i)) + (rpy_scale * thst_rpyt(i)); 
end

% Calculate throttle thrust after mixing for harmonic notch
thrOut = throttle_thrust_best_plus_adj / compGain;

% Assign thrust output
thstOut = thst_rpyt;

== matlab function arducopter/Position Controller/P Position z/Calculate error ==
  settings: updateMethod=DISCRETE
function [tar_new, err] = calc_err(tar, act, err_min, err_max)
% Code based on AC_P_1D::update_all() in AC_P_1D.cpp.
tar_new = tar; % added line to prevent Simulink error for unassigned tar_new
err = tar - act;

% Limit error and recalculate target
if ((err_min < 0) && (err < err_min))
    err = err_min;
    tar_new = act + err;
elseif ((err_max > 0) && (err > err_max))
    err = err_max;
    tar_new = act + err;
end
